simulink model "G3P3_Demo_2020a"  (R2023a)
settings: Solver=FixedStepAuto  StartTime=0.0  StopTime=86400  FixedStep=10  RelTol=1e-3
settings Model: Creator=Owner  LastModifiedBy=Owner
settings SolverCC: AlgebraicLoopSolver=TrustRegion

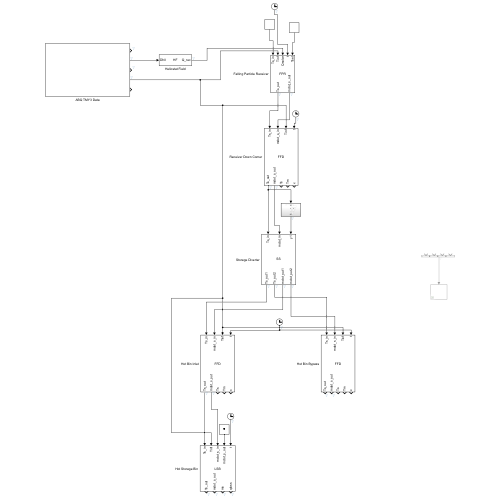
[thumbnail: Simulink's stored preview of the top-level diagram]
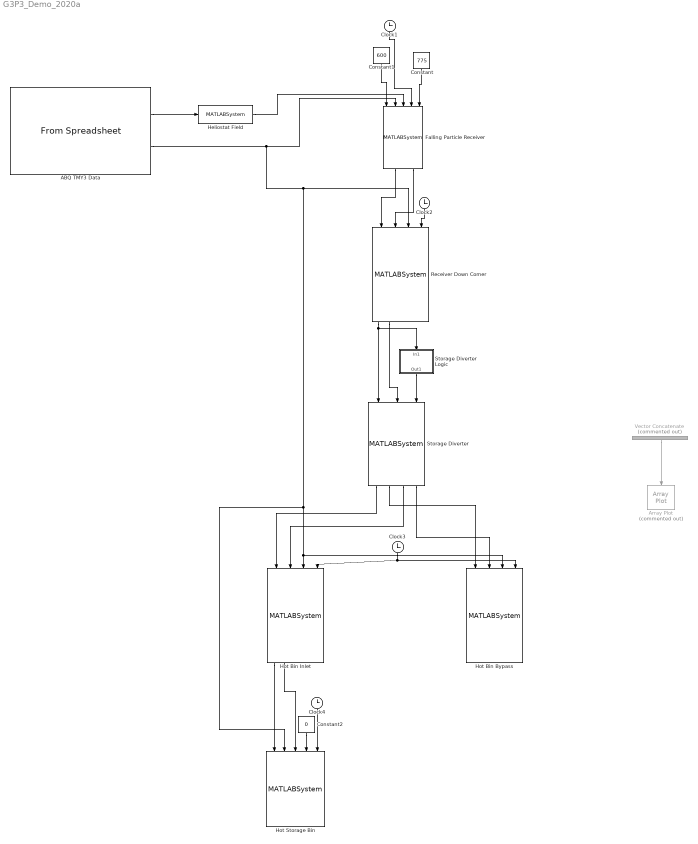
== system G3P3_Demo_2020a ==
  ABQ TMY3 Data : FromSpreadsheet  FileName=ABQ_Weather_Lookup.xlsx  OutDataTypeStr=double
  Array Plot : ArrayPlot  Commented=on  WindowPosition=[1014.000000,178.000000,800.000000,500.000000,]  YLimits=[-11.1356,100.2208]  ChannelNames=[']  DefaultConfigurationName=dsp.scopes.ArrayPlotBlockSpecification
  Clock{1..4} (4 alike) : Clock
  Constant : Constant  Value=775
  Constant1 : Constant  Value=600
  Constant2 : Constant  Value=0
  Falling Particle Receiver : MATLABSystem  System=FPR  H=1.2  W=1.2  d=0.0417  SimulateUsing=Code generation  Ts0=600  hInf=5  cp_s=1250  rho_s=3500  phi_s=0.6  epsilon_s=0.88  alpha_s=0.92  tauLag=1500  tauLead=100
      mask Type: FPR
      mask Display:
      | disp('FPR');
      | port_label('input',1,'Ts_in');
      | port_label('input',2,'Tinf');
      | port_label('input',3,'Qsolar');
      | port_label('input',4,'t');
      | port_label('input',5,'Tset');
      | port_label('output',1,'Ts_out');
      | port_label('output',2,'mdot_s_out');
  Heliostat Field : MATLABSystem  System=HF  n=150  H=5  W=5  eta_op=0.6  SimulateUsing=Code generation
      mask Type: HF
      mask Display:
      | disp('HF');
      | port_label('input',1,'DNI');
      | port_label('output',1,'Q_rec');
  Hot Bin Bypass : MATLABSystem  System=FFD  n=100  D=0.25  L=10  td=0.003  SimulateUsing=Code generation  Ts0=25  Tm0=25  cp_s=1250  rho_s=3500  phi_s=0.6  cp_m=500  rho_m=8000  hinf=10  hsw=100
      mask Type: FFD
      mask Display:
      | disp('FFD');
      | port_label('input',1,'Ts_in');
      | port_label('input',2,'mdot_s_in');
      | port_label('input',3,'Tinf');
      | port_label('input',4,'t');
      | port_label('output',1,'Ts_out');
      | port_label('output',2,'mdot_s_out');
      | port_label('output',3,'Ts');
      | port_label('output',4,'Tm');
      | port_label('output',5,'x');
  Hot Bin Inlet : MATLABSystem  System=FFD  n=100  D=0.25  L=10  td=0.003  SimulateUsing=Code generation  Ts0=25  Tm0=25  cp_s=1250  rho_s=3500  phi_s=0.6  cp_m=500  rho_m=8000  hinf=10  hsw=100
      mask Type: FFD
      mask Display:
      | disp('FFD');
      | port_label('input',1,'Ts_in');
      | port_label('input',2,'mdot_s_in');
      | port_label('input',3,'Tinf');
      | port_label('input',4,'t');
      | port_label('output',1,'Ts_out');
      | port_label('output',2,'mdot_s_out');
      | port_label('output',3,'Ts');
      | port_label('output',4,'Tm');
      | port_label('output',5,'x');
  Hot Storage Bin : MATLABSystem  System=LSB  H=7  D=5  SimulateUsing=Code generation  ms0=10  Ts0=615  ht=10  hinf=10  cp_s=1250  rho_s=3500  phi_s=0.98
      mask Type: LSB
      mask Display:
      | disp('LSB');
      | port_label('input',1,'Ts_in');
      | port_label('input',2,'Tinf');
      | port_label('input',3,'mdot_s_in');
      | port_label('input',4,'mdot_s_out');
      | port_label('input',5,'t');
      | port_label('output',1,'Ts_out');
      | port_label('output',2,'mdot_s_out');
      | port_label('output',3,'ms');
      | port_label('output',4,'qloss');
  Receiver Down Comer : MATLABSystem  System=FFD  n=100  D=0.25  L=10  td=0.003  SimulateUsing=Code generation  Ts0=25  Tm0=25  cp_s=1250  rho_s=3500  phi_s=0.6  cp_m=500  rho_m=8000  hinf=10  hsw=100
      mask Type: FFD
      mask Display:
      | disp('FFD');
      | port_label('input',1,'Ts_in');
      | port_label('input',2,'mdot_s_in');
      | port_label('input',3,'Tinf');
      | port_label('input',4,'t');
      | port_label('output',1,'Ts_out');
      | port_label('output',2,'mdot_s_out');
      | port_label('output',3,'Ts');
      | port_label('output',4,'Tm');
      | port_label('output',5,'x');
  Storage Diverter : MATLABSystem  System=SS  SimulateUsing=Code generation
      mask Type: SS
      mask Display:
      | disp('SS');
      | port_label('input',1,'Ts_in');
      | port_label('input',2,'mdot_in');
      | port_label('input',3,'y1');
      | port_label('output',1,'Ts_out1');
      | port_label('output',2,'Ts_out2');
      | port_label('output',3,'mdot_out1');
      | port_label('output',4,'mdot_out2');
  Storage Diverter Logic : Subsystem
  Vector Concatenate : Concatenate  Commented=on  NumInputs=4
  wires:
  ABQ TMY3 Data/4 -> Hot Storage Bin/2, Hot Bin Bypass/3, Hot Bin Inlet/3, Receiver Down Comer/3, Falling Particle Receiver/2
  ABQ TMY3 Data/2 -> Heliostat Field/1
  Clock1/1 -> Falling Particle Receiver/4
  Heliostat Field/1 -> Falling Particle Receiver/3
  Constant1/1 -> Falling Particle Receiver/1
  Constant/1 -> Falling Particle Receiver/5
  Vector Concatenate/1 -> Array Plot/1
  Falling Particle Receiver/1 -> Receiver Down Comer/1
  Falling Particle Receiver/2 -> Receiver Down Comer/2
  Clock2/1 -> Receiver Down Comer/4
  Receiver Down Comer/1 -> Storage Diverter Logic/1(In1), Storage Diverter/1
  Receiver Down Comer/2 -> Storage Diverter/2
  Storage Diverter Logic/1(Out1) -> Storage Diverter/3
  Storage Diverter/1 -> Hot Bin Inlet/1
  Storage Diverter/3 -> Hot Bin Inlet/2
  Clock3/1 -> Hot Bin Bypass/4, Hot Bin Inlet/4
  Storage Diverter/2 -> Hot Bin Bypass/1
  Storage Diverter/4 -> Hot Bin Bypass/2
  Hot Bin Inlet/1 -> Hot Storage Bin/1
  Hot Bin Inlet/2 -> Hot Storage Bin/3
  Clock4/1 -> Hot Storage Bin/5
  Constant2/1 -> Hot Storage Bin/4

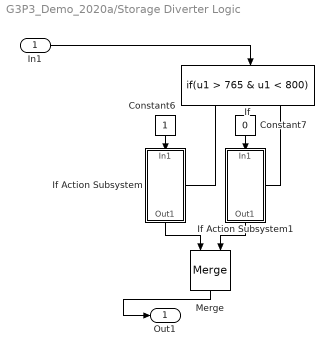
== system G3P3_Demo_2020a/Storage Diverter Logic ==
  In1 : Inport
  Constant6 : Constant
  Constant7 : Constant  Value=0
  If : If  IfExpression=u1 > 765 & u1 < 800
  If Action Subsystem : Subsystem  TreatAsAtomicUnit=on
  If Action Subsystem1 : Subsystem  TreatAsAtomicUnit=on
  Merge : Merge
  Out1 : Outport
  wires:
  If Action Subsystem1/1(Out1) -> Merge/2
  In1/1 -> If/1
  Constant6/1 -> If Action Subsystem/1(In1)
  Merge/1 -> Out1/1
  If Action Subsystem/1(Out1) -> Merge/1
  Constant7/1 -> If Action Subsystem1/1(In1)
  If/2 -> If Action Subsystem1/Action
  If/1 -> If Action Subsystem/Action

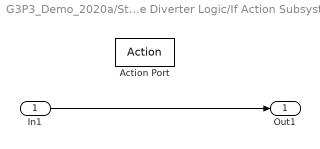
== system G3P3_Demo_2020a/Storage Diverter Logic/If Action Subsystem ==
  In1 : Inport
  Action Port : ActionPort  ActionPortLabel=if(u1 > 765 & u1 < 800)
  Out1 : Outport
  wires:
  In1/1 -> Out1/1

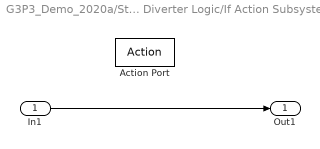
== system G3P3_Demo_2020a/Storage Diverter Logic/If Action Subsystem1 ==
  In1 : Inport
  Action Port : ActionPort  ActionPortLabel=else
  Out1 : Outport
  wires:
  In1/1 -> Out1/1
